simulink model "dofAutopilot3"  (R2024b)
settings: Solver=ode4  StartTime=0.0  StopTime=30  FixedStep=0.01  MaxStep=0.2  RelTol=1e-3
undefined symbols (not defined in the file or in its folder): aileron, AngulerRate, Attitude, BodyVelocities, elevator, rudder
libraries: slpidlib x5, shared6dof x1, simulink_extras x1
settings Model: Creator=sahil  LastModifiedBy=sahil

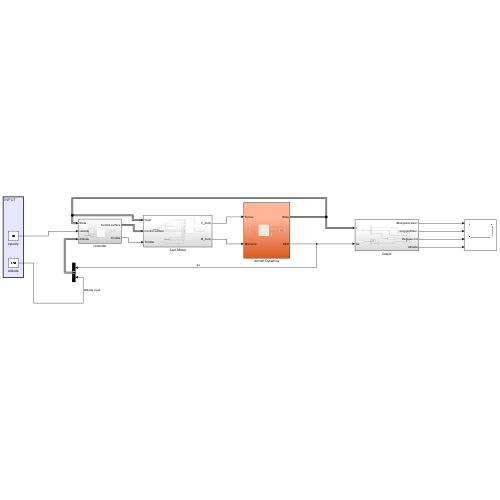
[thumbnail: Simulink's stored preview of the top-level diagram]
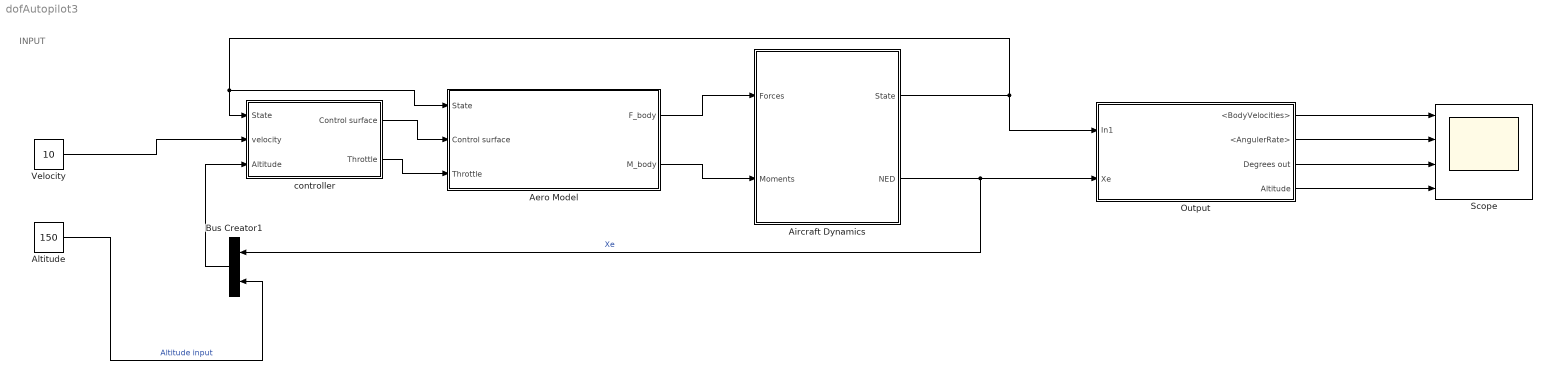
== system dofAutopilot3 ==
  note: INPUT
  Aero Model : Subsystem
  Aircraft Dynamics : Subsystem
  Altitude : Constant  Value=150
  Bus Creator1 : BusCreator  Inputs=Xe,Altitude input
  Output : Subsystem
  Scope : Scope  NumInputPorts=4
  Velocity : Constant  Value=10
  controller : Subsystem
  wires:
  Aero Model/1(F_body) -> Aircraft Dynamics/1(Forces)
  Aero Model/2(M_body) -> Aircraft Dynamics/2(Moments)
  controller/1(Control surface) -> Aero Model/2(Control surface)
  Velocity/1 -> controller/2(velocity)
  controller/2(Throttle) -> Aero Model/3(Throttle)
  Aircraft Dynamics/1(State) -> controller/1(State), Aero Model/1(State), Output/1(In1)
  Aircraft Dynamics/2(NED) -> Bus Creator1/1, Output/2(Xe)  "Xe"
  Altitude/1 -> Bus Creator1/2  "Altitude input"
  Bus Creator1/1 -> controller/3(Altitude)
  Output/1(<BodyVelocities>) -> Scope/1
  Output/2(<AngulerRate>) -> Scope/2
  Output/3(Degrees out) -> Scope/3
  Output/4(Altitude) -> Scope/4

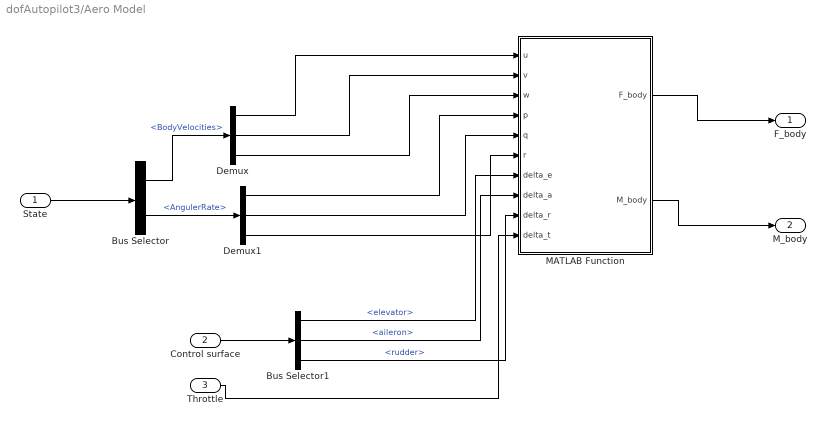
== system dofAutopilot3/Aero Model ==
  State : Inport
  Control surface : Inport  Port=2
  Throttle : Inport  Port=3
  Bus Selector : BusSelector  OutputSignals=BodyVelocities,AngulerRate
  Bus Selector1 : BusSelector  OutputSignals=elevator,aileron,rudder
  Demux : Demux  Outputs=3
  Demux1 : Demux  Outputs=3
  MATLAB Function : MATLAB Function  TreatAsAtomicUnit=on
  F_body : Outport
  M_body : Outport  Port=2
  wires:
  Bus Selector/2 -> Demux1/1  "<AngulerRate>"
  Demux1/3 -> MATLAB Function/6(r)
  Demux/1 -> MATLAB Function/1(u)
  Demux1/1 -> MATLAB Function/4(p)
  Demux/2 -> MATLAB Function/2(v)
  Demux/3 -> MATLAB Function/3(w)
  State/1 -> Bus Selector/1
  Demux1/2 -> MATLAB Function/5(q)
  Bus Selector/1 -> Demux/1  "<BodyVelocities>"
  MATLAB Function/2(M_body) -> M_body/1
  MATLAB Function/1(F_body) -> F_body/1
  Control surface/1 -> Bus Selector1/1
  Bus Selector1/1 -> MATLAB Function/7(delta_e)  "<elevator>"
  Bus Selector1/2 -> MATLAB Function/8(delta_a)  "<aileron>"
  Bus Selector1/3 -> MATLAB Function/9(delta_r)  "<rudder>"
  Throttle/1 -> MATLAB Function/10(delta_t)

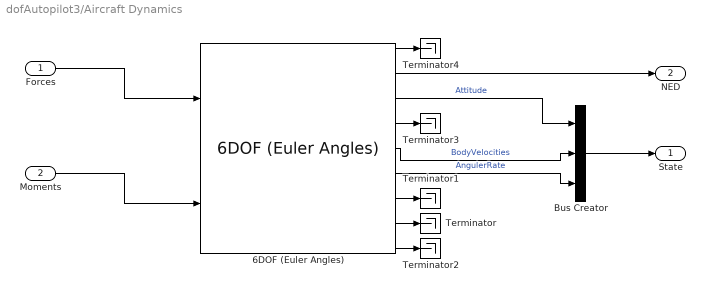
== system dofAutopilot3/Aircraft Dynamics ==
  Forces : Inport
  Moments : Inport  Port=2
  6DOF (Euler Angles) : shared6dof/6DOF (Euler Angles)  units=Metric (MKS)  mtype=Fixed  rep=Euler Angles  xme_0=[0 0 -100]  Vm_0=[0.1 0 0]  eul_0=[0 0 0]  pm_0=[0 0 0]  mass_0=m  mass_e=0.5  mass_f=2.0  inertia=I  inertia_e=eye(3)  inertia_f=2*eye(3)  k_quat=1.0  vre_flag=on  abi_flag=on  aMode=0  xme_statename=''  Vm_statename=''  eul_statename=''  quat_statename=''  pm_statename=''  mass_statename=''
  Bus Creator : BusCreator  Inputs=Attitude,BodyVelocities,AngulerRate
  Terminator{,1..4} (5 alike) : Terminator
  State : Outport
  NED : Outport  Port=2
  wires:
  6DOF (Euler Angles)/6 -> Bus Creator/3  "AngulerRate"
  6DOF (Euler Angles)/9 -> Terminator2/1
  6DOF (Euler Angles)/7 -> Terminator1/1
  6DOF (Euler Angles)/5 -> Bus Creator/2  "BodyVelocities"
  6DOF (Euler Angles)/8 -> Terminator/1
  Bus Creator/1 -> State/1
  Moments/1 -> 6DOF (Euler Angles)/2
  6DOF (Euler Angles)/1 -> Terminator4/1
  Forces/1 -> 6DOF (Euler Angles)/1
  6DOF (Euler Angles)/4 -> Terminator3/1
  6DOF (Euler Angles)/3 -> Bus Creator/1  "Attitude"
  6DOF (Euler Angles)/2 -> NED/1

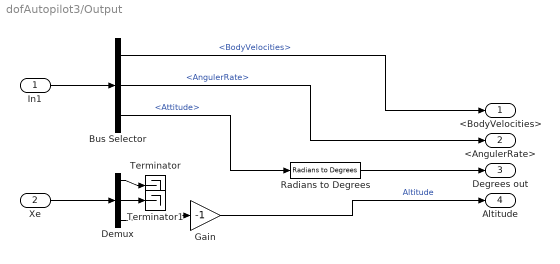
== system dofAutopilot3/Output ==
  In1 : Inport
  Xe : Inport  Port=2
  Bus Selector : BusSelector  OutputSignals=BodyVelocities,AngulerRate,Attitude
  Demux : Demux  Outputs=3
  Gain : Gain  Gain=-1
  Radians to Degrees : simulink_extras/Transformations/Radians to Degrees
  Terminator : Terminator
  Terminator1 : Terminator
  <BodyVelocities> : Outport
  <AngulerRate> : Outport  Port=2
  Degrees out : Outport  Port=3
  Altitude : Outport  Port=4
  wires:
  Demux/1 -> Terminator/1
  In1/1 -> Bus Selector/1
  Demux/3 -> Gain/1
  Demux/2 -> Terminator1/1
  Bus Selector/3 -> Radians to Degrees/1  "<Attitude>"
  Radians to Degrees/1 -> Degrees out/1
  Gain/1 -> Altitude/1  "Altitude"
  Xe/1 -> Demux/1
  Bus Selector/1 -> <BodyVelocities>/1  "<BodyVelocities>"
  Bus Selector/2 -> <AngulerRate>/1  "<AngulerRate>"

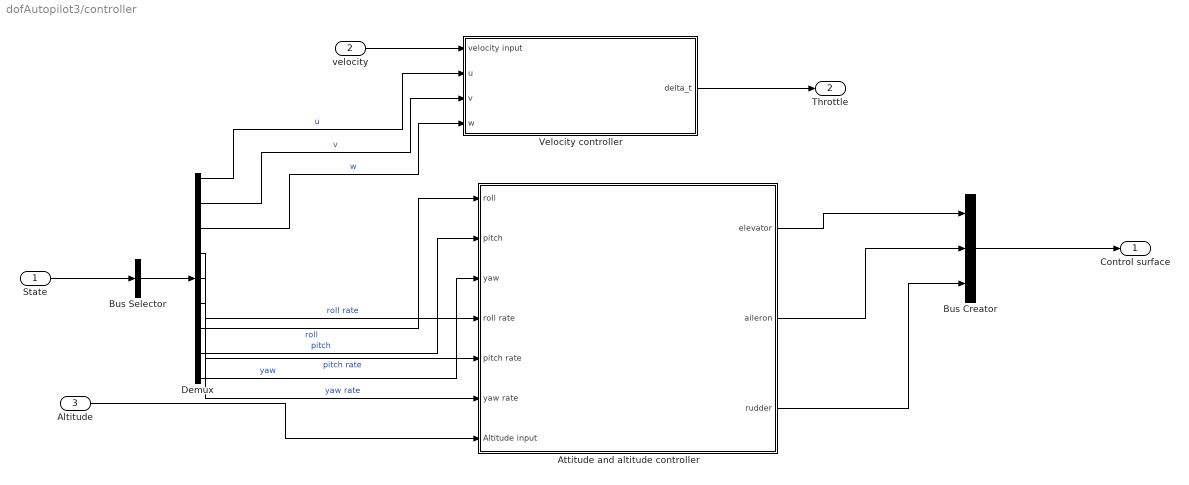
== system dofAutopilot3/controller ==
  State : Inport
  velocity : Inport  Port=2
  Altitude : Inport  Port=3
  Attitude and altitude controller : Subsystem
  Bus Creator : BusCreator  Inputs=elevator,aileron,rudder
  Bus Selector : BusSelector  OutputSignals=BodyVelocities,AngulerRate,Attitude  OutputAsBus=on
  Demux : Demux  Outputs=9
  Velocity controller : Subsystem
  Control surface : Outport
  Throttle : Outport  Port=2
  wires:
  State/1 -> Bus Selector/1
  Bus Selector/1 -> Demux/1
  Bus Creator/1 -> Control surface/1
  Demux/4 -> Attitude and altitude controller/4(roll rate)  "roll rate"
  Demux/5 -> Attitude and altitude controller/5(pitch rate)  "pitch rate"
  Demux/6 -> Attitude and altitude controller/6(yaw rate)  "yaw rate"
  Attitude and altitude controller/1(elevator) -> Bus Creator/1
  Attitude and altitude controller/2(aileron) -> Bus Creator/2
  Attitude and altitude controller/3(rudder) -> Bus Creator/3
  Demux/7 -> Attitude and altitude controller/1(roll)  "roll"
  Demux/8 -> Attitude and altitude controller/2(pitch)  "pitch"
  Demux/9 -> Attitude and altitude controller/3(yaw)  "yaw"
  velocity/1 -> Velocity controller/1(velocity input)
  Demux/1 -> Velocity controller/2(u)  "u"
  Demux/2 -> Velocity controller/3(v)  "v"
  Demux/3 -> Velocity controller/4(w)  "w"
  Velocity controller/1(delta_t) -> Throttle/1
  Altitude/1 -> Attitude and altitude controller/7(Altitude input)

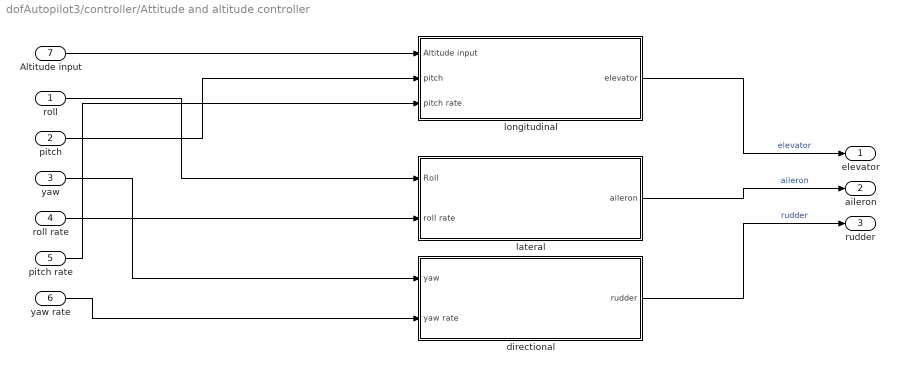
== system dofAutopilot3/controller/Attitude and altitude controller ==
  roll : Inport
  pitch : Inport  Port=2
  yaw : Inport  Port=3
  roll rate : Inport  Port=4
  pitch rate : Inport  Port=5
  yaw rate : Inport  Port=6
  Altitude input : Inport  Port=7
  directional : Subsystem
  lateral : Subsystem
  longitudinal : Subsystem
  elevator : Outport
  aileron : Outport  Port=2
  rudder : Outport  Port=3
  wires:
  roll/1 -> lateral/1(Roll)
  pitch/1 -> longitudinal/2(pitch)
  yaw/1 -> directional/1(yaw)
  longitudinal/1(elevator) -> elevator/1  "elevator"
  yaw rate/1 -> directional/2(yaw rate)
  roll rate/1 -> lateral/2(roll rate)
  directional/1(rudder) -> rudder/1  "rudder"
  lateral/1(aileron) -> aileron/1  "aileron"
  pitch rate/1 -> longitudinal/3(pitch rate)
  Altitude input/1 -> longitudinal/1(Altitude input)

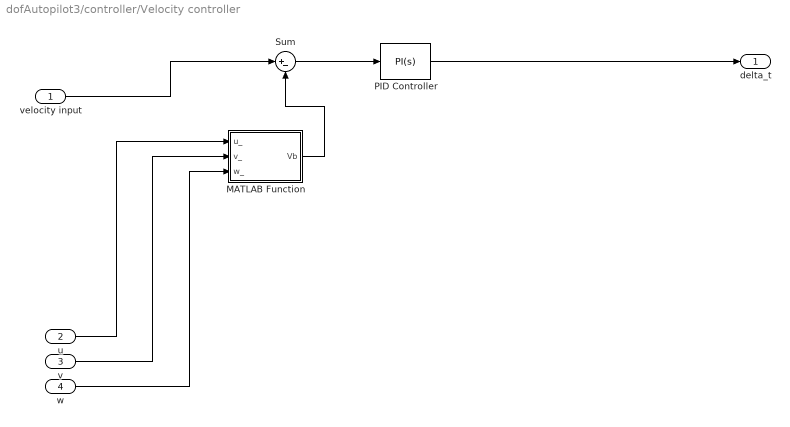
== system dofAutopilot3/controller/Velocity controller ==
  velocity input : Inport
  u : Inport  Port=2
  v : Inport  Port=3
  w : Inport  Port=4
  MATLAB Function : MATLAB Function  TreatAsAtomicUnit=on
  PID Controller : slpidlib/PID Controller  Controller=PI  Form=Parallel  TimeDomain=Continuous-time  UseExternalTs=off  SampleTime=-1  IntegratorMethod=Forward Euler  FilterMethod=Forward Euler  ControllerParametersSource=internal  P=0.1  I=0.05  UseKiTs=off  D=0  UseExternalDerivativeSource=off  N=100  UseFilter=on  TunerSelectOption=Transfer Function Based (PID Tuner App)  InitialConditionSource=internal  InitialConditionForIntegrator=0  InitialConditionForFilter=0  DifferentiatorICPrevScaledInput=0  ExternalReset=none  TrackingMode=off  Kt=1  LimitOutput=on  SatLimitsSource=internal  UpperSaturationLimit=1  LowerSaturationLimit=0  LinearizeAsGain=on  AntiWindupMode=none  Kb=1  LimitIntegrator=off  UpperIntegratorSaturationLimit=inf  LowerIntegratorSaturationLimit=-inf  POutMin=[]  POutMax=[]  IOutMin=[]  IOutMax=[]  DOutMin=[]  DOutMax=[]  NOutMin=[]  NOutMax=[]  SumOutMin=[]  SumOutMax=[]  SaturationOutMin=[]  SaturationOutMax=[]  PParamMin=[]  PParamMax=[]  IParamMin=[]  IParamMax=[]  DParamMin=[]  DParamMax=[]  NParamMin=[]  NParamMax=[]  KbParamMin=[]  KbParamMax=[]  KtParamMin=[]  KtParamMax=[]  KbOutMin=[]  KbOutMax=[]  KtOutMin=[]  KtOutMax=[]  IntegratorOutMin=[]  IntegratorOutMax=[]  FilterOutMin=[]  FilterOutMax=[]  SumI1OutMin=[]  SumI1OutMax=[]  SumI2OutMin=[]  SumI2OutMax=[]  SumI3OutMin=[]  SumI3OutMax=[]  SumI4OutMin=[]  SumI4OutMax=[]  SumDOutMin=[]  SumDOutMax=[]  DifferentiatorOutMin=[]  DifferentiatorOutMax=[]  FilterDiffOutCoefMin=[]  FilterDiffOutCoefMax=[]  ReciprocalOutMin=[]  ReciprocalOutMax=[]  SumDenOutMin=[]  SumDenOutMax=[]  SumNumOutMin=[]  SumNumOutMax=[]  DivideOutMin=[]  DivideOutMax=[]  UdiffTsProdOutMin=[]  UdiffTsProdOutMax=[]  NTsProdOutMin=[]  NTsProdOutMax=[]  UintegralTsProdOutMin=[]  UintegralTsProdOutMax=[]  UngainTsProdOutMin=[]  UngainTsProdOutMax=[]  ClampingZeroOutDataTypeStr=Inherit: Inherit via back propagation  ClampingZeroOutMin=[]  ClampingZeroOutMax=[]  FilterDenConstantOutDataTypeStr=Inherit: Inherit via back propagation  FilterDenConstantOutMin=[]  FilterDenConstantOutMax=[]  PCopyOutDataTypeStr=Inherit: Inherit via back propagation  PCopyOutMin=[]  PCopyOutMax=[]  NCopyOutDataTypeStr=Inherit: Inherit via back propagation  NCopyOutMin=[]  NCopyOutMax=[]  IntegratorContinuousStateAttributes=''  IntegratorStateMustResolveToSignalObject=off  IntegratorRTWStateStorageClass=Auto  FilterContinuousStateAttributes=''  FilterStateMustResolveToSignalObject=off  FilterRTWStateStorageClass=Auto  ParallelPVariant=InternalParameters  IdealPVariant=Disabled  IVariant=InternalParameters  DVariant=Disabled  IntegratorVariant=Continuous  SatVariant=Enabled  AWVariant=Passthrough  PCopyVariant=Disabled  TRVariant=Disabled  FdbkBlocksVariant=Forward  IdealPFdbkVariant=Disabled  SatFdbkVariant=Disabled  DerivativeFilterVariant=Disabled  NVariant=Disabled  NCopyVariant=Disabled_SignalSpec  FilterICVariant=Disabled  IntegratorICVariant=InternalICs  ExternalResetVariant=Disabled  TRSumVariant=Passthrough  SumFdbkVariant=Disabled  SumVariant=Sum_PI  TsampFilterVariant=InternalTs  TsampNgainVariant=Passthrough  TsampIntegralVariant=Disabled_SignalSpec  ExternalSaturationOutDataTypeStr=Inherit: Same as second input  DerivativeSourceVariant=Disabled  PreIntVariant=InternalPreInt
  Sum : Sum  Inputs=|+-
  delta_t : Outport
  wires:
  PID Controller/1 -> delta_t/1
  Sum/1 -> PID Controller/1
  MATLAB Function/1(Vb) -> Sum/2
  u/1 -> MATLAB Function/1(u_)
  velocity input/1 -> Sum/1
  w/1 -> MATLAB Function/3(w_)
  v/1 -> MATLAB Function/2(v_)

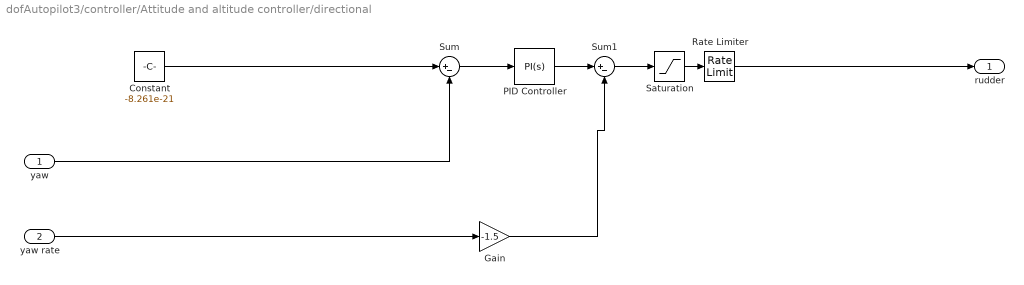
== system dofAutopilot3/controller/Attitude and altitude controller/directional ==
  yaw : Inport
  yaw rate : Inport  Port=2
  Constant : Constant  Value=-8.261e-21  VectorParams1D=off
  Gain : Gain  Gain=-1.5
  PID Controller : slpidlib/PID Controller  Controller=PI  Form=Parallel  TimeDomain=Continuous-time  UseExternalTs=off  SampleTime=-1  IntegratorMethod=Forward Euler  FilterMethod=Forward Euler  ControllerParametersSource=internal  P=-1.2  I=-4.2  UseKiTs=on  D=0  UseExternalDerivativeSource=off  N=100  UseFilter=on  TunerSelectOption=Transfer Function Based (PID Tuner App)  InitialConditionSource=internal  InitialConditionForIntegrator=0  InitialConditionForFilter=0  DifferentiatorICPrevScaledInput=0  ExternalReset=none  TrackingMode=off  Kt=1  LimitOutput=off  SatLimitsSource=internal  UpperSaturationLimit=inf  LowerSaturationLimit=-inf  LinearizeAsGain=on  AntiWindupMode=none  Kb=1  LimitIntegrator=off  UpperIntegratorSaturationLimit=inf  LowerIntegratorSaturationLimit=-inf  POutMin=[]  POutMax=[]  IOutMin=[]  IOutMax=[]  DOutMin=[]  DOutMax=[]  NOutMin=[]  NOutMax=[]  SumOutMin=[]  SumOutMax=[]  SaturationOutMin=[]  SaturationOutMax=[]  PParamMin=[]  PParamMax=[]  IParamMin=[]  IParamMax=[]  DParamMin=[]  DParamMax=[]  NParamMin=[]  NParamMax=[]  KbParamMin=[]  KbParamMax=[]  KtParamMin=[]  KtParamMax=[]  KbOutMin=[]  KbOutMax=[]  KtOutMin=[]  KtOutMax=[]  IntegratorOutMin=[]  IntegratorOutMax=[]  FilterOutMin=[]  FilterOutMax=[]  SumI1OutMin=[]  SumI1OutMax=[]  SumI2OutMin=[]  SumI2OutMax=[]  SumI3OutMin=[]  SumI3OutMax=[]  SumI4OutMin=[]  SumI4OutMax=[]  SumDOutMin=[]  SumDOutMax=[]  DifferentiatorOutMin=[]  DifferentiatorOutMax=[]  FilterDiffOutCoefMin=[]  FilterDiffOutCoefMax=[]  ReciprocalOutMin=[]  ReciprocalOutMax=[]  SumDenOutMin=[]  SumDenOutMax=[]  SumNumOutMin=[]  SumNumOutMax=[]  DivideOutMin=[]  DivideOutMax=[]  UdiffTsProdOutMin=[]  UdiffTsProdOutMax=[]  NTsProdOutMin=[]  NTsProdOutMax=[]  UintegralTsProdOutMin=[]  UintegralTsProdOutMax=[]  UngainTsProdOutMin=[]  UngainTsProdOutMax=[]  ClampingZeroOutDataTypeStr=Inherit: Inherit via back propagation  ClampingZeroOutMin=[]  ClampingZeroOutMax=[]  FilterDenConstantOutDataTypeStr=Inherit: Inherit via back propagation  FilterDenConstantOutMin=[]  FilterDenConstantOutMax=[]  PCopyOutDataTypeStr=Inherit: Inherit via back propagation  PCopyOutMin=[]  PCopyOutMax=[]  NCopyOutDataTypeStr=Inherit: Inherit via back propagation  NCopyOutMin=[]  NCopyOutMax=[]  IntegratorContinuousStateAttributes=''  IntegratorStateMustResolveToSignalObject=off  IntegratorRTWStateStorageClass=Auto  FilterContinuousStateAttributes=''  FilterStateMustResolveToSignalObject=off  FilterRTWStateStorageClass=Auto  ParallelPVariant=InternalParameters  IdealPVariant=Disabled  IVariant=InternalParameters  DVariant=Disabled  IntegratorVariant=Continuous  SatVariant=Disabled  AWVariant=Passthrough  PCopyVariant=Disabled  TRVariant=Disabled  FdbkBlocksVariant=Forward  IdealPFdbkVariant=Disabled  SatFdbkVariant=Disabled  DerivativeFilterVariant=Disabled  NVariant=Disabled  NCopyVariant=Disabled_SignalSpec  FilterICVariant=Disabled  IntegratorICVariant=InternalICs  ExternalResetVariant=Disabled  TRSumVariant=Passthrough  SumFdbkVariant=Disabled  SumVariant=Sum_PI  TsampFilterVariant=InternalTs  TsampNgainVariant=Passthrough  TsampIntegralVariant=Disabled_SignalSpec  ExternalSaturationOutDataTypeStr=Inherit: Same as second input  DerivativeSourceVariant=Disabled  PreIntVariant=InternalPreInt
  Rate Limiter : RateLimiter  RisingSlewLimit=60/57.3  FallingSlewLimit=-60/57.3  SampleTimeMode=inherited
  Saturation : Saturate  UpperLimit=30/57.3  LowerLimit=-30/57.3
  Sum : Sum  Inputs=|+-
  Sum1 : Sum  Inputs=|+-
  rudder : Outport
  wires:
  Sum1/1 -> Saturation/1
  yaw/1 -> Sum/2
  PID Controller/1 -> Sum1/1
  Sum/1 -> PID Controller/1
  Saturation/1 -> Rate Limiter/1
  yaw rate/1 -> Gain/1
  Gain/1 -> Sum1/2
  Constant/1 -> Sum/1
  Rate Limiter/1 -> rudder/1

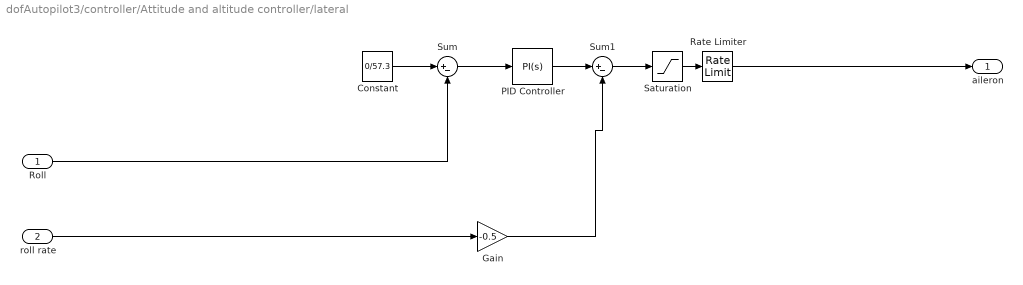
== system dofAutopilot3/controller/Attitude and altitude controller/lateral ==
  Roll : Inport
  roll rate : Inport  Port=2
  Constant : Constant  Value=0/57.3
  Gain : Gain  Gain=-0.5
  PID Controller : slpidlib/PID Controller  Controller=PI  Form=Parallel  TimeDomain=Continuous-time  UseExternalTs=off  SampleTime=-1  IntegratorMethod=Forward Euler  FilterMethod=Forward Euler  ControllerParametersSource=internal  P=-0.8  I=-0.45  UseKiTs=on  D=0  UseExternalDerivativeSource=off  N=100  UseFilter=on  TunerSelectOption=Transfer Function Based (PID Tuner App)  InitialConditionSource=internal  InitialConditionForIntegrator=0  InitialConditionForFilter=0  DifferentiatorICPrevScaledInput=0  ExternalReset=none  TrackingMode=off  Kt=1  LimitOutput=off  SatLimitsSource=internal  UpperSaturationLimit=inf  LowerSaturationLimit=-inf  LinearizeAsGain=on  AntiWindupMode=none  Kb=1  LimitIntegrator=off  UpperIntegratorSaturationLimit=inf  LowerIntegratorSaturationLimit=-inf  POutMin=[]  POutMax=[]  IOutMin=[]  IOutMax=[]  DOutMin=[]  DOutMax=[]  NOutMin=[]  NOutMax=[]  SumOutMin=[]  SumOutMax=[]  SaturationOutMin=[]  SaturationOutMax=[]  PParamMin=[]  PParamMax=[]  IParamMin=[]  IParamMax=[]  DParamMin=[]  DParamMax=[]  NParamMin=[]  NParamMax=[]  KbParamMin=[]  KbParamMax=[]  KtParamMin=[]  KtParamMax=[]  KbOutMin=[]  KbOutMax=[]  KtOutMin=[]  KtOutMax=[]  IntegratorOutMin=[]  IntegratorOutMax=[]  FilterOutMin=[]  FilterOutMax=[]  SumI1OutMin=[]  SumI1OutMax=[]  SumI2OutMin=[]  SumI2OutMax=[]  SumI3OutMin=[]  SumI3OutMax=[]  SumI4OutMin=[]  SumI4OutMax=[]  SumDOutMin=[]  SumDOutMax=[]  DifferentiatorOutMin=[]  DifferentiatorOutMax=[]  FilterDiffOutCoefMin=[]  FilterDiffOutCoefMax=[]  ReciprocalOutMin=[]  ReciprocalOutMax=[]  SumDenOutMin=[]  SumDenOutMax=[]  SumNumOutMin=[]  SumNumOutMax=[]  DivideOutMin=[]  DivideOutMax=[]  UdiffTsProdOutMin=[]  UdiffTsProdOutMax=[]  NTsProdOutMin=[]  NTsProdOutMax=[]  UintegralTsProdOutMin=[]  UintegralTsProdOutMax=[]  UngainTsProdOutMin=[]  UngainTsProdOutMax=[]  ClampingZeroOutDataTypeStr=Inherit: Inherit via back propagation  ClampingZeroOutMin=[]  ClampingZeroOutMax=[]  FilterDenConstantOutDataTypeStr=Inherit: Inherit via back propagation  FilterDenConstantOutMin=[]  FilterDenConstantOutMax=[]  PCopyOutDataTypeStr=Inherit: Inherit via back propagation  PCopyOutMin=[]  PCopyOutMax=[]  NCopyOutDataTypeStr=Inherit: Inherit via back propagation  NCopyOutMin=[]  NCopyOutMax=[]  IntegratorContinuousStateAttributes=''  IntegratorStateMustResolveToSignalObject=off  IntegratorRTWStateStorageClass=Auto  FilterContinuousStateAttributes=''  FilterStateMustResolveToSignalObject=off  FilterRTWStateStorageClass=Auto  ParallelPVariant=InternalParameters  IdealPVariant=Disabled  IVariant=InternalParameters  DVariant=Disabled  IntegratorVariant=Continuous  SatVariant=Disabled  AWVariant=Passthrough  PCopyVariant=Disabled  TRVariant=Disabled  FdbkBlocksVariant=Forward  IdealPFdbkVariant=Disabled  SatFdbkVariant=Disabled  DerivativeFilterVariant=Disabled  NVariant=Disabled  NCopyVariant=Disabled_SignalSpec  FilterICVariant=Disabled  IntegratorICVariant=InternalICs  ExternalResetVariant=Disabled  TRSumVariant=Passthrough  SumFdbkVariant=Disabled  SumVariant=Sum_PI  TsampFilterVariant=InternalTs  TsampNgainVariant=Passthrough  TsampIntegralVariant=Disabled_SignalSpec  ExternalSaturationOutDataTypeStr=Inherit: Same as second input  DerivativeSourceVariant=Disabled  PreIntVariant=InternalPreInt
  Rate Limiter : RateLimiter  RisingSlewLimit=20/57.3  FallingSlewLimit=-20/57.3  SampleTimeMode=inherited
  Saturation : Saturate  UpperLimit=25/57.3  LowerLimit=-25/57.3
  Sum : Sum  Inputs=|+-
  Sum1 : Sum  Inputs=|+-
  aileron : Outport
  wires:
  Rate Limiter/1 -> aileron/1
  Gain/1 -> Sum1/2
  roll rate/1 -> Gain/1
  Saturation/1 -> Rate Limiter/1
  Sum/1 -> PID Controller/1
  PID Controller/1 -> Sum1/1
  Roll/1 -> Sum/2
  Sum1/1 -> Saturation/1
  Constant/1 -> Sum/1

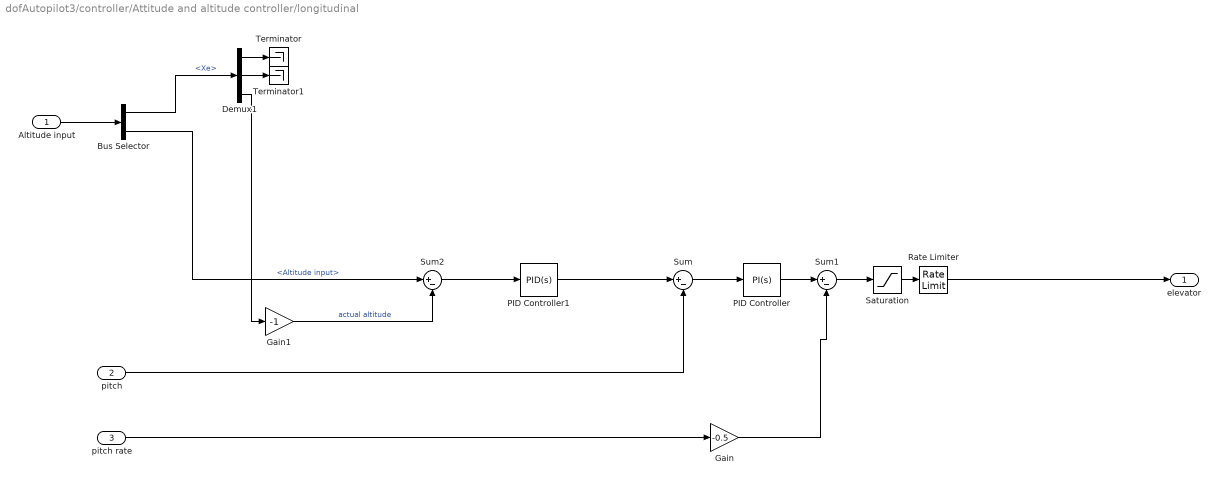
== system dofAutopilot3/controller/Attitude and altitude controller/longitudinal ==
  Altitude input : Inport
  pitch : Inport  Port=2
  pitch rate : Inport  Port=3
  Bus Selector : BusSelector  OutputSignals=Xe,Altitude input
  Demux1 : Demux  Outputs=3
  Gain : Gain  Gain=-0.5
  Gain1 : Gain  Gain=-1
  PID Controller : slpidlib/PID Controller  Controller=PI  Form=Parallel  TimeDomain=Continuous-time  UseExternalTs=off  SampleTime=-1  IntegratorMethod=Forward Euler  FilterMethod=Forward Euler  ControllerParametersSource=internal  P=-0.8  I=-0.45  UseKiTs=on  D=0  UseExternalDerivativeSource=off  N=100  UseFilter=on  TunerSelectOption=Transfer Function Based (PID Tuner App)  InitialConditionSource=internal  InitialConditionForIntegrator=0  InitialConditionForFilter=0  DifferentiatorICPrevScaledInput=0  ExternalReset=none  TrackingMode=off  Kt=1  LimitOutput=off  SatLimitsSource=internal  UpperSaturationLimit=inf  LowerSaturationLimit=-inf  LinearizeAsGain=on  AntiWindupMode=none  Kb=1  LimitIntegrator=off  UpperIntegratorSaturationLimit=inf  LowerIntegratorSaturationLimit=-inf  POutMin=[]  POutMax=[]  IOutMin=[]  IOutMax=[]  DOutMin=[]  DOutMax=[]  NOutMin=[]  NOutMax=[]  SumOutMin=[]  SumOutMax=[]  SaturationOutMin=[]  SaturationOutMax=[]  PParamMin=[]  PParamMax=[]  IParamMin=[]  IParamMax=[]  DParamMin=[]  DParamMax=[]  NParamMin=[]  NParamMax=[]  KbParamMin=[]  KbParamMax=[]  KtParamMin=[]  KtParamMax=[]  KbOutMin=[]  KbOutMax=[]  KtOutMin=[]  KtOutMax=[]  IntegratorOutMin=[]  IntegratorOutMax=[]  FilterOutMin=[]  FilterOutMax=[]  SumI1OutMin=[]  SumI1OutMax=[]  SumI2OutMin=[]  SumI2OutMax=[]  SumI3OutMin=[]  SumI3OutMax=[]  SumI4OutMin=[]  SumI4OutMax=[]  SumDOutMin=[]  SumDOutMax=[]  DifferentiatorOutMin=[]  DifferentiatorOutMax=[]  FilterDiffOutCoefMin=[]  FilterDiffOutCoefMax=[]  ReciprocalOutMin=[]  ReciprocalOutMax=[]  SumDenOutMin=[]  SumDenOutMax=[]  SumNumOutMin=[]  SumNumOutMax=[]  DivideOutMin=[]  DivideOutMax=[]  UdiffTsProdOutMin=[]  UdiffTsProdOutMax=[]  NTsProdOutMin=[]  NTsProdOutMax=[]  UintegralTsProdOutMin=[]  UintegralTsProdOutMax=[]  UngainTsProdOutMin=[]  UngainTsProdOutMax=[]  ClampingZeroOutDataTypeStr=Inherit: Inherit via back propagation  ClampingZeroOutMin=[]  ClampingZeroOutMax=[]  FilterDenConstantOutDataTypeStr=Inherit: Inherit via back propagation  FilterDenConstantOutMin=[]  FilterDenConstantOutMax=[]  PCopyOutDataTypeStr=Inherit: Inherit via back propagation  PCopyOutMin=[]  PCopyOutMax=[]  NCopyOutDataTypeStr=Inherit: Inherit via back propagation  NCopyOutMin=[]  NCopyOutMax=[]  IntegratorContinuousStateAttributes=''  IntegratorStateMustResolveToSignalObject=off  IntegratorRTWStateStorageClass=Auto  FilterContinuousStateAttributes=''  FilterStateMustResolveToSignalObject=off  FilterRTWStateStorageClass=Auto  ParallelPVariant=InternalParameters  IdealPVariant=Disabled  IVariant=InternalParameters  DVariant=Disabled  IntegratorVariant=Continuous  SatVariant=Disabled  AWVariant=Passthrough  PCopyVariant=Disabled  TRVariant=Disabled  FdbkBlocksVariant=Forward  IdealPFdbkVariant=Disabled  SatFdbkVariant=Disabled  DerivativeFilterVariant=Disabled  NVariant=Disabled  NCopyVariant=Disabled_SignalSpec  FilterICVariant=Disabled  IntegratorICVariant=InternalICs  ExternalResetVariant=Disabled  TRSumVariant=Passthrough  SumFdbkVariant=Disabled  SumVariant=Sum_PI  TsampFilterVariant=InternalTs  TsampNgainVariant=Passthrough  TsampIntegralVariant=Disabled_SignalSpec  ExternalSaturationOutDataTypeStr=Inherit: Same as second input  DerivativeSourceVariant=Disabled  PreIntVariant=InternalPreInt
  PID Controller1 : slpidlib/PID Controller  Controller=PID  Form=Parallel  TimeDomain=Continuous-time  UseExternalTs=off  SampleTime=-1  IntegratorMethod=Forward Euler  FilterMethod=Forward Euler  ControllerParametersSource=internal  P=0.04  I=0  UseKiTs=off  D=0.08  UseExternalDerivativeSource=off  N=100  UseFilter=on  TunerSelectOption=Transfer Function Based (PID Tuner App)  InitialConditionSource=internal  InitialConditionForIntegrator=0  InitialConditionForFilter=0  DifferentiatorICPrevScaledInput=0  ExternalReset=none  TrackingMode=off  Kt=1  LimitOutput=on  SatLimitsSource=internal  UpperSaturationLimit=25/57.3  LowerSaturationLimit=-25/57.3  LinearizeAsGain=on  AntiWindupMode=none  Kb=1  LimitIntegrator=off  UpperIntegratorSaturationLimit=inf  LowerIntegratorSaturationLimit=-inf  POutMin=[]  POutMax=[]  IOutMin=[]  IOutMax=[]  DOutMin=[]  DOutMax=[]  NOutMin=[]  NOutMax=[]  SumOutMin=[]  SumOutMax=[]  SaturationOutMin=[]  SaturationOutMax=[]  PParamMin=[]  PParamMax=[]  IParamMin=[]  IParamMax=[]  DParamMin=[]  DParamMax=[]  NParamMin=[]  NParamMax=[]  KbParamMin=[]  KbParamMax=[]  KtParamMin=[]  KtParamMax=[]  KbOutMin=[]  KbOutMax=[]  KtOutMin=[]  KtOutMax=[]  IntegratorOutMin=[]  IntegratorOutMax=[]  FilterOutMin=[]  FilterOutMax=[]  SumI1OutMin=[]  SumI1OutMax=[]  SumI2OutMin=[]  SumI2OutMax=[]  SumI3OutMin=[]  SumI3OutMax=[]  SumI4OutMin=[]  SumI4OutMax=[]  SumDOutMin=[]  SumDOutMax=[]  DifferentiatorOutMin=[]  DifferentiatorOutMax=[]  FilterDiffOutCoefMin=[]  FilterDiffOutCoefMax=[]  ReciprocalOutMin=[]  ReciprocalOutMax=[]  SumDenOutMin=[]  SumDenOutMax=[]  SumNumOutMin=[]  SumNumOutMax=[]  DivideOutMin=[]  DivideOutMax=[]  UdiffTsProdOutMin=[]  UdiffTsProdOutMax=[]  NTsProdOutMin=[]  NTsProdOutMax=[]  UintegralTsProdOutMin=[]  UintegralTsProdOutMax=[]  UngainTsProdOutMin=[]  UngainTsProdOutMax=[]  ClampingZeroOutDataTypeStr=Inherit: Inherit via back propagation  ClampingZeroOutMin=[]  ClampingZeroOutMax=[]  FilterDenConstantOutDataTypeStr=Inherit: Inherit via back propagation  FilterDenConstantOutMin=[]  FilterDenConstantOutMax=[]  PCopyOutDataTypeStr=Inherit: Inherit via back propagation  PCopyOutMin=[]  PCopyOutMax=[]  NCopyOutDataTypeStr=Inherit: Inherit via back propagation  NCopyOutMin=[]  NCopyOutMax=[]  IntegratorContinuousStateAttributes=''  IntegratorStateMustResolveToSignalObject=off  IntegratorRTWStateStorageClass=Auto  FilterContinuousStateAttributes=''  FilterStateMustResolveToSignalObject=off  FilterRTWStateStorageClass=Auto  ParallelPVariant=InternalParameters  IdealPVariant=Disabled  IVariant=InternalParameters  DVariant=InternalParameters  IntegratorVariant=Continuous  SatVariant=Enabled  AWVariant=Passthrough  PCopyVariant=Disabled  TRVariant=Disabled  FdbkBlocksVariant=Forward  IdealPFdbkVariant=Disabled  SatFdbkVariant=Disabled  DerivativeFilterVariant=ContFilter  NVariant=InternalParameters  NCopyVariant=Disabled  FilterICVariant=InternalICsFilter  IntegratorICVariant=InternalICs  ExternalResetVariant=Disabled  TRSumVariant=Passthrough  SumFdbkVariant=Disabled  SumVariant=Sum_PID  TsampFilterVariant=InternalTs  TsampNgainVariant=Passthrough  TsampIntegralVariant=Disabled_SignalSpec  ExternalSaturationOutDataTypeStr=Inherit: Same as second input  DerivativeSourceVariant=ErrorSignal  PreIntVariant=InternalPreInt
  Rate Limiter : RateLimiter  RisingSlewLimit=20/57.3  FallingSlewLimit=-20/57.3  SampleTimeMode=inherited
  Saturation : Saturate  UpperLimit=25/57.3  LowerLimit=-25/57.3
  Sum : Sum  Inputs=|+-
  Sum1 : Sum  Inputs=|+-
  Sum2 : Sum  Inputs=|+-
  Terminator : Terminator
  Terminator1 : Terminator
  elevator : Outport
  wires:
  Sum1/1 -> Saturation/1
  pitch/1 -> Sum/2
  PID Controller/1 -> Sum1/1
  Sum/1 -> PID Controller/1
  Saturation/1 -> Rate Limiter/1
  pitch rate/1 -> Gain/1
  Gain/1 -> Sum1/2
  Rate Limiter/1 -> elevator/1
  Sum2/1 -> PID Controller1/1
  Altitude input/1 -> Bus Selector/1
  Demux1/3 -> Gain1/1
  Demux1/2 -> Terminator1/1
  Demux1/1 -> Terminator/1
  Bus Selector/1 -> Demux1/1  "<Xe>"
  Bus Selector/2 -> Sum2/1  "<Altitude input>"
  Gain1/1 -> Sum2/2  "actual altitude"
  PID Controller1/1 -> Sum/1

== matlab function dofAutopilot3/controller/Velocity controller/MATLAB Function ==
  data: u_ input; Vb output; v_ input; w_ input
function Vb = fcn(u_,v_,w_)

Vb = sqrt((u_)^2+(v_)^2+(w_)^2);
end

== matlab function dofAutopilot3/Aero Model/MATLAB Function ==
  data: u input; F_body output; v input; w input; p input; q input; r input; M_body output; delta_e input; delta_a input; delta_r input; delta_t input
function [F_body, M_body] = Aero(u, v, w, p, q, r, delta_e, delta_a, delta_r, delta_t)

% ==========================================================
% 1. GEOMETRY & ENVIRONMENT
% ==========================================================
rho = 1.225;     % Air density (kg/m^3)
S   = 0.5;       % Wing area (m^2)
b   = 2.0;       % Wingspan (m)
c   = 0.25;      % Mean aerodynamic chord (m)
T_max = 250;


% ==========================================================
% 2. NON-DIMENSIONAL AERODYNAMIC DERIVATIVES
% ==========================================================

% --- Longitudinal Derivatives ---
CL0   = 0.3;     % Lift at zero alpha
CLa   = 4.5;     % Lift curve slope (per rad)
CD0   = 0.03;    % Parasitic drag
K_drg = 0.3;     % Induced drag factor (CD = CD0 + K*alpha^2)

Cm0   = 0.0;     % Pitching moment at zero alpha
Cma   = -0.5;    % Pitch static stability
Cmq   = -8.0;    % Pitch damping
Cmde  = -1.2;    % Elevator control effectiveness

% --- Lateral-Directional Derivatives ---
CYb   = -0.98;   % Side force due to sideslip
CYdr  = 0.15;    % Side force due to rudder

Clb   = -0.12;   % Dihedral effect (Roll due to sideslip)
Clp   = -0.5;    % Roll damping
Clr   = 0.0;     % Roll due to yaw rate (Cross-derivative)
Clda  = -0.15;   % Aileron control effectiveness
Cldr  = 0.0;     % Roll due to rudder (Cross-derivative)

Cnb   = 0.25;    % Weathercock stability (Yaw due to sideslip)
Cnp   = 0.0;     % Yaw due to roll rate (Cross-derivative)
Cnr   = -0.3;    % Yaw damping
Cnda  = 0.0;     % Yaw due to aileron (Adverse yaw)
Cndr  = -0.1;    % Rudder control effectiveness

% ==========================================================
% 3. KINEMATIC STATE VARIABLES
% ==========================================================
V = sqrt(u^2 + v^2 + w^2);
if V < 0.1
    V = 0.1; % Prevent division by zero at initialization
end

alpha = atan2(w, u);     % Angle of attack (rad)
beta  = asin(v / V);     % Sideslip angle (rad)
q_bar = 0.5 * rho * V^2; % Dynamic pressure (N/m^2)

% Non-dimensional angular rates
p_hat = (p * b) / (2 * V);
q_hat = (q * c) / (2 * V);
r_hat = (r * b) / (2 * V);

% ==========================================================
% 4. TOTAL AERODYNAMIC COEFFICIENTS
% ==========================================================
% Lift and Drag (Simplified parabolic drag polar)
CL = CL0 + (CLa * alpha);
CD = CD0 + (K_drg * alpha^2);

% Side Force
CY = (CYb * beta) + (CYdr * delta_r);

% Rolling Moment
Cl = (Clb * beta) + (Clp * p_hat) + (Clr * r_hat) + (Clda * delta_a) + (Cldr * delta_r);

% Pitching Moment
Cm = Cm0 + (Cma * alpha) + (Cmq * q_hat) + (Cmde * delta_e);

% Yawing Moment
Cn = (Cnb * beta) + (Cnp * p_hat) + (Cnr * r_hat) + (Cnda * delta_a) + (Cndr * delta_r);

% ==========================================================
% 5. DIMENSIONAL FORCES (BODY FRAME)
% ==========================================================
% Convert wind frame (Lift/Drag) to body frame (Fx, Fz)
Fx = (T_max * delta_t) - CD * q_bar * S * cos(alpha) + CL * q_bar * S * sin(alpha);
Fz = -CD * q_bar * S * sin(alpha) - CL * q_bar * S * cos(alpha);
Fy = CY * q_bar * S;

F_body = [Fx; Fy; Fz];

% ==========================================================
% 6. DIMENSIONAL MOMENTS (BODY FRAME)
% ==========================================================
Mx = Cl * q_bar * S * b;
My = Cm * q_bar * S * c;
Mz = Cn * q_bar * S * b;

M_body = [Mx; My; Mz];

end
